simulink model "THE_ACTUAL_regulator"  (R2024a)
settings: Solver=VariableStepAuto  StartTime=0.0  StopTime=5  MaxStep=1e-3  RelTol=1e-3
values from neighbouring files (symbols this model uses):
  F = F_e(:, 1:4)    [split_F.m]
  FI = F_e(:, 5:6)    [split_FI.m]
  sys_init = randn([4 1])    [sim_vars.m]
undefined symbols (not defined in the file or in its folder): A, B, C, L
settings Model: Creator=kasper  LastModifiedBy=balder
settings RTWCC: GPUComputeCapability=3.5

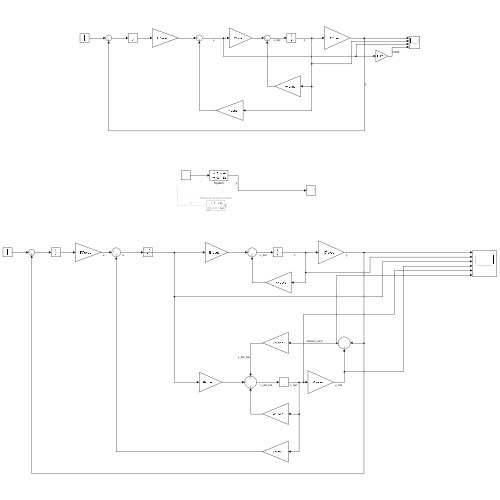
[thumbnail: Simulink's stored preview of the top-level diagram]
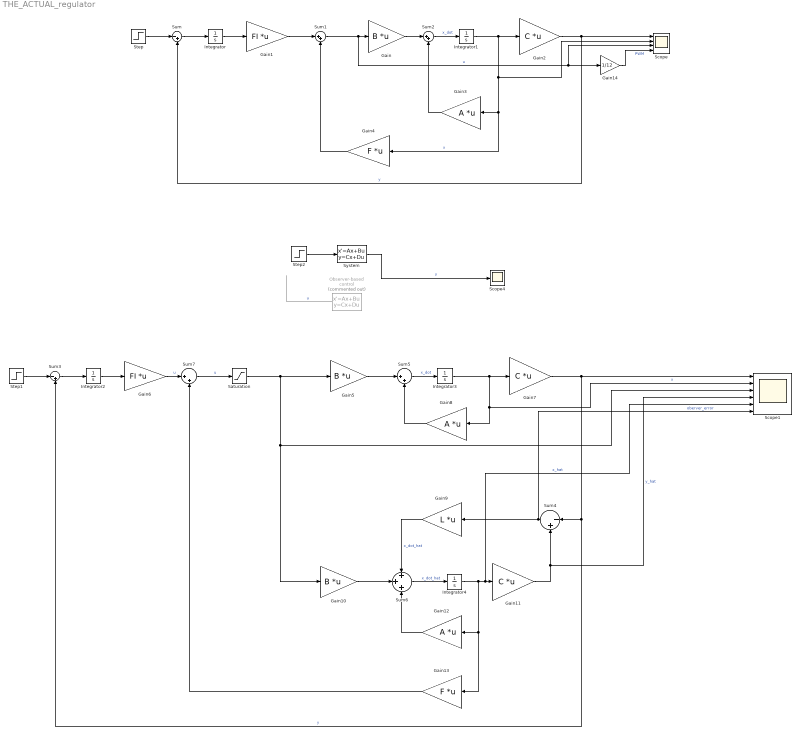
== system THE_ACTUAL_regulator ==
  Gain : Gain  Gain=B  Multiplication=Matrix(K*u) (u vector)
  Gain1 : Gain  Gain=FI  Multiplication=Matrix(K*u) (u vector)
  Gain10 : Gain  Gain=B  Multiplication=Matrix(K*u) (u vector)
  Gain11 : Gain  Gain=C  Multiplication=Matrix(K*u) (u vector)
  Gain12 : Gain  Gain=A  Multiplication=Matrix(K*u) (u vector)
  Gain13 : Gain  Gain=F  Multiplication=Matrix(K*u) (u vector)
  Gain14 : Gain  Gain=1/12
  Gain2 : Gain  Gain=C  Multiplication=Matrix(K*u) (u vector)
  Gain3 : Gain  Gain=A  Multiplication=Matrix(K*u) (u vector)
  Gain4 : Gain  Gain=F  Multiplication=Matrix(K*u) (u vector)
  Gain5 : Gain  Gain=B  Multiplication=Matrix(K*u) (u vector)
  Gain6 : Gain  Gain=FI  Multiplication=Matrix(K*u) (u vector)
  Gain7 : Gain  Gain=C  Multiplication=Matrix(K*u) (u vector)
  Gain8 : Gain  Gain=A  Multiplication=Matrix(K*u) (u vector)
  Gain9 : Gain  Gain=L  Multiplication=Matrix(K*u) (u vector)
  Integrator : Integrator
  Integrator1 : Integrator
  Integrator2 : Integrator
  Integrator3 : Integrator  InitialCondition=sys_init
  Integrator4 : Integrator  UpperSaturationLimit=100  LowerSaturationLimit=-100
  Observer-based control : StateSpace  Commented=on  A=A+B*F+L*C  B=-L  C=F  D=zeros(2)  InitialCondition=0
  Saturation : Saturate  UpperLimit=12  LowerLimit=-12
  Scope : Scope  NumInputPorts=4
  Scope1 : Scope  NumInputPorts=6
  Scope4 : Scope
  Step : Step  Before=[0 0]  After=[1 1]  SampleTime=0
  Step1 : Step  Time=2  Before=[0 0]  After=[1 2]  SampleTime=0
  Step2 : Step  Before=[-1; -1]  After=[0; 0]  SampleTime=0
  Sum : Sum  Inputs=|-+
  Sum{1..2,5,7} (4 alike) : Sum  Inputs=|++
  Sum3 : Sum  Inputs=|-+
  Sum4 : Sum  Inputs=|-+
  Sum6 : Sum  Inputs=+++
  System : StateSpace  A=A  B=B  C=C  D=zeros(2)  InitialCondition=0
  wires:
  Step/1 -> Sum/1
  Sum/1 -> Integrator/1
  Integrator/1 -> Gain1/1
  Gain1/1 -> Sum1/1
  Sum1/1 -> Scope/3, Gain14/1, Gain/1  "u"
  Gain/1 -> Sum2/1
  Sum2/1 -> Integrator1/1  "x_dot"
  Integrator1/1 -> Gain4/1, Gain3/1, Scope/2, Gain2/1  "x"
  Gain3/1 -> Sum2/2
  Gain4/1 -> Sum1/2
  Gain2/1 -> Sum/2, Scope/1  "y"
  Integrator3/1 -> Gain8/1, Scope1/2, Gain7/1  "x"
  Sum7/1 -> Saturation/1  "u"
  Step1/1 -> Sum3/1
  Gain8/1 -> Sum5/2
  Gain5/1 -> Sum5/1
  Sum3/1 -> Integrator2/1
  Integrator2/1 -> Gain6/1
  Sum5/1 -> Integrator3/1  "x_dot"
  Gain7/1 -> Sum4/1, Sum3/2, Scope1/1  "y"
  Sum4/1 -> Scope1/6, Gain9/1  "oberver_error"
  Gain10/1 -> Sum6/2
  Sum6/1 -> Integrator4/1  "x_dot_hat"
  Integrator4/1 -> Gain11/1, Scope1/5, Gain13/1, Gain12/1  "x_hat"
  Gain11/1 -> Scope1/4, Sum4/2  "y_hat"
  Gain12/1 -> Sum6/3
  Gain13/1 -> Sum7/2
  System/1 -> Scope4/1  "y"
  Observer-based control/1 -> ?  "u"
  Gain6/1 -> Sum7/1  "u"
  Step2/1 -> System/1
  Gain14/1 -> Scope/4  "PWM"
  Gain9/1 -> Sum6/1  "x_dot_hat"
  Saturation/1 -> Gain5/1, Gain10/1, Scope1/3
